simulink model "sampleModel2432_pp_1_1"  (R2018a)
settings: Solver=VariableStepAuto  StartTime=0.0  StopTime=10.0  RelTol=1e-3
undefined symbols (not defined in the file or in its folder): DiscIntNeverNeededParam, sigbuilder_block
libraries: simulink x293
(part 1 of 7)
settings Model: Creator=cyfuzz  LastModifiedBy=ishaf
settings CodeAppCC: StateflowObjectComments=on

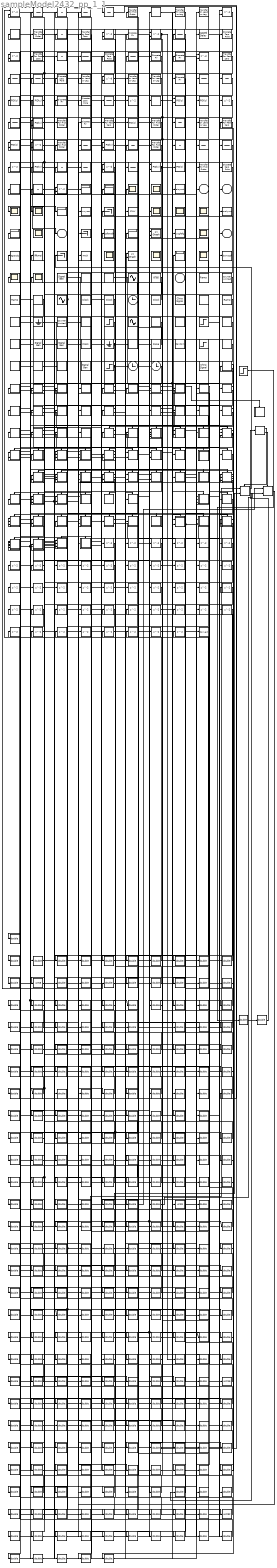
== system sampleModel2432_pp_1_1 ==
  cfblk128 : Inport
  cfblk{1,10,15,17,21,62,83} (7 alike) : Delay  ShowEnablePort=on  SampleTime=1
      settings: InputPortMap=u0,e6
  cfblk100 : ToWorkspace  VariableName=sxokymd  SaveFormat=Timeseries  SampleTime=-1
  cfblk{84..85,93,101,106,118} (6 alike) : Display
  cfblk{86..87,91..92,97..99,102,109,115,117,119,121..122} (14 alike) : Scope
      cfblk102 settings: Floating=on
      cfblk109 settings: Floating=on
      cfblk115 settings: Floating=on
      cfblk117 settings: Floating=on
      cfblk119 settings: Floating=on
      cfblk87 settings: Floating=on
      cfblk98 settings: Floating=on
      cfblk99 settings: Floating=on
  cfblk104 : Terminator
  cfblk105 : ToWorkspace  VariableName=zdioxsb  SaveFormat=Timeseries  SampleTime=-1
  cfblk107 : simulink/Sinks/XY Graph  xmin=-1  xmax=1  ymin=-1  ymax=1  st=-1
  cfblk108 : ToWorkspace  VariableName=yqgfefg  SaveFormat=Timeseries  SampleTime=-1
  cfblk11 : DiscreteStateSpace
  cfblk111 : ToWorkspace  VariableName=egcazdz  SaveFormat=Timeseries  SampleTime=-1
  cfblk112 : ToWorkspace  VariableName=iffcmsi  SaveFormat=Timeseries  SampleTime=-1
  cfblk113 : Terminator
  cfblk114 : ToFile  Filename=nxck  SaveFormat=Timeseries
  cfblk116 : simulink/Sinks/XY Graph  xmin=-1  xmax=1  ymin=-1  ymax=1  st=-1
  cfblk{6,12,53,57,63,67,79} (7 alike) : simulink/Discrete/Transfer Fcn First Order  PoleZ=0.95  ICPrevOutput=0.0  DoSatur=off
      settings: SourceProductName=Simulink
  cfblk120 : ToWorkspace  VariableName=bomsczf  SaveFormat=Timeseries  SampleTime=-1
  cfblk{123,152..153,164} (4 alike) : SignalGenerator  Units=rad/sec
  cfblk{124..125,132,139,147,163} (6 alike) : simulink/Sources/Repeating Sequence Interpolated  OutValues=[3 1 4 2 1].'  TimeValues=[0 0.1 0.5 0.6 1].'  LookUpMeth=Interpolation-Use End Values  tsamp=0.01  OutMin=[]  OutMax=[]  OutDataTypeStr=double  OutputDataTypeScalingMode=double  OutDataType=fixdt(0,8)  OutScaling=2^-10
  cfblk126 : Sin  SampleTime=0
  cfblk127 : Constant  Value=8785
  cfblk129 : simulink/Sources/Ramp  slope=1  start=0  InitialOutput=0
  cfblk{3,13,23,68,73,82} (6 alike) : UnitDelay
  cfblk130 : simulink/Sources/Counter Limited  uplimit=7  tsamp=-1
  cfblk131 : simulink/Sources/Ramp  slope=1  start=0  InitialOutput=0
  cfblk133 : Sin  SampleTime=0
  cfblk{134..135,137,154} (4 alike) : DigitalClock
  cfblk136 : Clock
  cfblk138 : simulink/Sources/Chirp Signal  f1=0.1  T=100  f2=1
  cfblk{14,22,30,55,60} (5 alike) : simulink/Discrete/Transfer Fcn Real Zero  ZeroZ=0.75  ICPrevInput=0.0  DoSatur=off
      settings: SourceProductName=Simulink  SourceProductBaseCode=SL
  cfblk140 : simulink/Sources/Ramp  slope=1  start=0  InitialOutput=0
  cfblk141 : Subsystem  Tag=STV Subsys  LoadFcn=sigbuilder_block('load');  StartFcn=sigbuilder_block('start');  StopFcn=sigbuilder_block('stop');  ClipboardFcn=sigbuilder_block('clipboard');  mask(Sigbuilder block){tuvar=[0:10]}
      mask help: Simulink:masks:SigbuilderBlock_MD
      mask init:
      | if ~strcmp(get_param(bdroot(gcbh),'SimulationStatus'),'stopped') tuvar = sigbuilder_block('maskInit'); end
      settings: CopyFcn=sigbuilder_block('copy');  DeleteFcn=sigbuilder_block('delete');  ModelCloseFcn=sigbuilder_block('modelClose');  PreSaveFcn=sigbuilder_block('preSave');  PauseFcn=sigbuilder_block('pause');  ContinueFcn=sigbuilder_block('continue');  NameChangeFcn=sigbuilder_block('namechange');  OpenFcn=sigbuilder_block('open',[437.6 199.2 550.4 400 ]);  CloseFcn=sigbuilder_block('close');
      mask Display: plot(0, 0, 100, 100,[2, 2, 32, 32, 2], [68, 8, 8, 68, 68],[32, 2], [38, 38], [32, 19, 2],[53, 60, 44], [32, 17, 17, 2],[16, 16, 31, 31]);txt = getActiveGroup(gcbh);text(2, 100, txt,'verticalAlignment', 'top');
  cfblk142 : Ground
  cfblk143 : simulink/Sources/Counter Limited  uplimit=7  tsamp=-1
  cfblk{144,150,160..161} (4 alike) : simulink/Sources/Repeating Sequence  rep_seq_t=[0 2]  rep_seq_y=[0 2]
  cfblk145 : Step  After=94  SampleTime=0
  cfblk146 : Sin  SampleTime=0
  cfblk148 : simulink/Sources/Repeating Sequence Stair  OutValues=[3 1 4 2 1].'  tsamp=-1  OutMin=[]  OutMax=[]  OutDataTypeStr=double  OutputDataTypeScalingMode=double  OutDataType=fixdt(0,8)  ConRadixGroup=Best Precision: Vector-wise  OutScaling=2^-12
  cfblk149 : Step  After=59  SampleTime=0
  cfblk151 : simulink/Sources/Band-Limited White Noise  Cov=[0.1]  Ts=0.1  seed=[23341]
  cfblk155 : Ground
  cfblk156 : Subsystem  Tag=STV Subsys  LoadFcn=sigbuilder_block('load');  StartFcn=sigbuilder_block('start');  StopFcn=sigbuilder_block('stop');  ClipboardFcn=sigbuilder_block('clipboard');  mask(Sigbuilder block){tuvar=[0:10]}
      mask help: Simulink:masks:SigbuilderBlock_MD
      mask init:
      | if ~strcmp(get_param(bdroot(gcbh),'SimulationStatus'),'stopped') tuvar = sigbuilder_block('maskInit'); end
      settings: CopyFcn=sigbuilder_block('copy');  DeleteFcn=sigbuilder_block('delete');  ModelCloseFcn=sigbuilder_block('modelClose');  PreSaveFcn=sigbuilder_block('preSave');  PauseFcn=sigbuilder_block('pause');  ContinueFcn=sigbuilder_block('continue');  NameChangeFcn=sigbuilder_block('namechange');  OpenFcn=sigbuilder_block('open',[437.6 199.2 550.4 400 ]);  CloseFcn=sigbuilder_block('close');
      mask Display: plot(0, 0, 100, 100,[2, 2, 32, 32, 2], [68, 8, 8, 68, 68],[32, 2], [38, 38], [32, 19, 2],[53, 60, 44], [32, 17, 17, 2],[16, 16, 31, 31]);txt = getActiveGroup(gcbh);text(2, 100, txt,'verticalAlignment', 'top');
  cfblk157 : DiscretePulseGenerator  PulseType=Time based  Period=10  PulseWidth=5
  cfblk158 : UniformRandomNumber  SampleTime=0.1
  cfblk159 : Step  After=53  SampleTime=0
  cfblk{16,27..28,38,43,54} (6 alike) : DiscreteFir  SampleTime=1
  cfblk162 : simulink/Sources/Counter Free-Running  NumBits=16  tsamp=-1
  cfblk165 : Step  After=66  SampleTime=0
  cfblk166 : Clock
  cfblk167 : Clock
  cfblk168 : Step  After=29  SampleTime=0
  cfblk169 : simulink/Sources/Chirp Signal  f1=0.1  T=100  f2=1
  cfblk{170..194} (25 alike) : If  SampleTime=1
  cfblk{2,18,51,64,70,74} (6 alike) : DiscreteTransferFcn  SampleTime=1
  cfblk19 : simulink/Discrete/Tapped Delay  vinit=0.0  samptime=-1  NumDelays=1  DelayOrder=Oldest  includeCurrent=off
  cfblk195 : Subsystem  TreatAsAtomicUnit=on
  cfblk196 : Subsystem  TreatAsAtomicUnit=on
  cfblk197 : Subsystem  TreatAsAtomicUnit=on
  cfblk198 : Subsystem  TreatAsAtomicUnit=on
  cfblk199 : Subsystem  TreatAsAtomicUnit=on
  cfblk{20,25,33,44,80} (5 alike) : DiscreteZeroPole  Poles=[0 0.5]  Gain=1
  cfblk200 : Subsystem  TreatAsAtomicUnit=on
  cfblk201 : Subsystem  TreatAsAtomicUnit=on
  cfblk202 : Subsystem  TreatAsAtomicUnit=on
  cfblk203 : Subsystem  TreatAsAtomicUnit=on
  cfblk204 : Subsystem  TreatAsAtomicUnit=on
  cfblk205 : Subsystem  TreatAsAtomicUnit=on
  cfblk206 : Subsystem  TreatAsAtomicUnit=on
  cfblk207 : Subsystem  TreatAsAtomicUnit=on
  cfblk208 : Subsystem  TreatAsAtomicUnit=on
  cfblk209 : Subsystem  TreatAsAtomicUnit=on
  cfblk210 : Subsystem  TreatAsAtomicUnit=on
  cfblk211 : Subsystem  TreatAsAtomicUnit=on
  cfblk212 : Subsystem  TreatAsAtomicUnit=on
  cfblk213 : Subsystem  TreatAsAtomicUnit=on
  cfblk214 : Subsystem  TreatAsAtomicUnit=on
  cfblk215 : Subsystem  TreatAsAtomicUnit=on
  cfblk216 : Subsystem  TreatAsAtomicUnit=on
  cfblk217 : Subsystem  TreatAsAtomicUnit=on
  cfblk218 : Subsystem  TreatAsAtomicUnit=on
  cfblk219 : Subsystem  TreatAsAtomicUnit=on
  cfblk220 : Subsystem  TreatAsAtomicUnit=on
  cfblk221 : Subsystem  TreatAsAtomicUnit=on
  cfblk222 : Subsystem  TreatAsAtomicUnit=on
  cfblk223 : Subsystem  TreatAsAtomicUnit=on
  cfblk224 : Subsystem  TreatAsAtomicUnit=on
  cfblk225 : Subsystem  TreatAsAtomicUnit=on
  cfblk226 : Subsystem  TreatAsAtomicUnit=on
  cfblk227 : Subsystem  TreatAsAtomicUnit=on
  cfblk228 : Subsystem  TreatAsAtomicUnit=on
  cfblk229 : Subsystem  TreatAsAtomicUnit=on
  cfblk230 : Subsystem  TreatAsAtomicUnit=on
  cfblk231 : Subsystem  TreatAsAtomicUnit=on
  cfblk232 : Subsystem  TreatAsAtomicUnit=on
  cfblk233 : Subsystem  TreatAsAtomicUnit=on
  cfblk234 : Subsystem  TreatAsAtomicUnit=on
  cfblk235 : Subsystem  TreatAsAtomicUnit=on
  cfblk236 : Subsystem  TreatAsAtomicUnit=on
  cfblk237 : Subsystem  TreatAsAtomicUnit=on
  cfblk238 : Subsystem  TreatAsAtomicUnit=on
  cfblk239 : Subsystem  TreatAsAtomicUnit=on
  cfblk{24,26,31..32,39,45,76} (7 alike) : DiscreteFilter  SampleTime=1
  cfblk240 : Subsystem  TreatAsAtomicUnit=on
  cfblk241 : Subsystem  TreatAsAtomicUnit=on
  cfblk242 : Subsystem  TreatAsAtomicUnit=on
  cfblk243 : Subsystem  TreatAsAtomicUnit=on
  cfblk244 : Subsystem  TreatAsAtomicUnit=on
  cfblk{46,50,71,245..288} (47 alike) : Delay  SampleTime=1
  cfblk289 : DataTypeConversion
  cfblk29 : Delay  DelayLengthSource=Input port  SampleTime=1
      settings: InputPortMap=u0,p1
  cfblk{8..9,34,36..37,59} (6 alike) : simulink/Discrete/Transfer Fcn Lead or Lag  PoleZ=0.95  ZeroZ=0.75  ICPrevOutput=0.0  ICPrevInput=0.0  DoSatur=off
      settings: SourceProductName=Simulink  SourceProductBaseCode=SL
  cfblk35 : Delay  DelayLengthSource=Input port  SampleTime=1
      settings: InputPortMap=u0,p1
  cfblk{4..5,40,58,66,69} (6 alike) : DiscreteIntegrator  ICPrevOutput=DiscIntNeverNeededParam  ICPrevScaledInput=DiscIntNeverNeededParam
  cfblk{41..42,49,56,72,78} (6 alike) : simulink/Continuous/PID Controller  Controller=PID  TimeDomain=Discrete-time  SampleTime=1  IntegratorMethod=Forward Euler  FilterMethod=Forward Euler  Form=Parallel  UseFilter=on  ControllerParametersSource=internal  P=1  I=1  D=0  N=100  InitialConditionSource=internal  InitialConditionForIntegrator=0  InitialConditionForFilter=0  ExternalReset=none  LimitOutput=off  UpperSaturationLimit=inf  LowerSaturationLimit=-inf  LinearizeAsGain=off  AntiWindupMode=none  Kb=1  TrackingMode=off  Kt=1  PParamMin=[]  PParamMax=[]  IParamMin=[]  IParamMax=[]  DParamMin=[]  DParamMax=[]  NParamMin=[]  NParamMax=[]  KbParamMin=[]  KbParamMax=[]  KtParamMin=[]  KtParamMax=[]  POutMin=[]  POutMax=[]  IOutMin=[]  IOutMax=[]  DOutMin=[]  DOutMax=[]  NOutMin=[]  NOutMax=[]  KbOutMin=[]  KbOutMax=[]  KtOutMin=[]  KtOutMax=[]  IntegratorOutMin=[]  IntegratorOutMax=[]  FilterOutMin=[]  FilterOutMax=[]  SumOutMin=[]  SumOutMax=[]  SumI1OutMin=[]  SumI1OutMax=[]  SumI2OutMin=[]  SumI2OutMax=[]  SumI3OutMin=[]  SumI3OutMax=[]  SumDOutMin=[]  SumDOutMax=[]  SaturationOutMin=[]  SaturationOutMax=[]  IntegratorContinuousStateAttributes=''  IntegratorStateMustResolveToSignalObject=off  IntegratorRTWStateStorageClass=Auto  FilterContinuousStateAttributes=''  FilterStateMustResolveToSignalObject=off  FilterRTWStateStorageClass=Auto  DifferentiatorICPrevScaledInput=0  DifferentiatorOutMin=[]  DifferentiatorOutMax=[]  FilterDiffOutCoefMin=[]  FilterDiffOutCoefMax=[]  SumDenOutMin=[]  SumDenOutMax=[]  SumNumOutMin=[]  SumNumOutMax=[]  ReciprocalOutMin=[]  ReciprocalOutMax=[]  DivideOutMin=[]  DivideOutMax=[]  TunerSelectOption=Transfer Function Based (PID Tuner App)
  cfblk47 : DiscreteStateSpace
  cfblk{48,52,61,65,77} (5 alike) : simulink/Continuous/PID Controller (2DOF)  Controller=PID  TimeDomain=Discrete-time  SampleTime=1  IntegratorMethod=Forward Euler  FilterMethod=Forward Euler  Form=Parallel  UseFilter=on  ControllerParametersSource=internal  P=1  I=1  D=0  N=100  b=1  c=1  InitialConditionSource=internal  InitialConditionForIntegrator=0  InitialConditionForFilter=0  ExternalReset=none  LimitOutput=off  UpperSaturationLimit=inf  LowerSaturationLimit=-inf  LinearizeAsGain=off  AntiWindupMode=none  Kb=1  TrackingMode=off  Kt=1  PParamMin=[]  PParamMax=[]  IParamMin=[]  IParamMax=[]  DParamMin=[]  DParamMax=[]  NParamMin=[]  NParamMax=[]  bParamMin=[]  bParamMax=[]  cParamMin=[]  cParamMax=[]  KbParamMin=[]  KbParamMax=[]  KtParamMin=[]  KtParamMax=[]  POutMin=[]  POutMax=[]  IOutMin=[]  IOutMax=[]  DOutMin=[]  DOutMax=[]  NOutMin=[]  NOutMax=[]  bOutMin=[]  bOutMax=[]  cOutMin=[]  cOutMax=[]  KbOutMin=[]  KbOutMax=[]  KtOutMin=[]  KtOutMax=[]  IntegratorOutMin=[]  IntegratorOutMax=[]  FilterOutMin=[]  FilterOutMax=[]  SumOutMin=[]  SumOutMax=[]  Sum1OutMin=[]  Sum1OutMax=[]  Sum2OutMin=[]  Sum2OutMax=[]  Sum3OutMin=[]  Sum3OutMax=[]  SumI1OutMin=[]  SumI1OutMax=[]  SumI2OutMin=[]  SumI2OutMax=[]  SumI3OutMin=[]  SumI3OutMax=[]  SumDOutMin=[]  SumDOutMax=[]  SaturationOutMin=[]  SaturationOutMax=[]  IntegratorContinuousStateAttributes=''  IntegratorStateMustResolveToSignalObject=off  IntegratorRTWStateStorageClass=Auto  FilterContinuousStateAttributes=''  FilterStateMustResolveToSignalObject=off  FilterRTWStateStorageClass=Auto  DifferentiatorICPrevScaledInput=0  DifferentiatorOutMin=[]  DifferentiatorOutMax=[]  FilterDiffOutCoefMin=[]  FilterDiffOutCoefMax=[]  SumDenOutMin=[]  SumDenOutMax=[]  SumNumOutMin=[]  SumNumOutMax=[]  ReciprocalOutMin=[]  ReciprocalOutMax=[]  DivideOutMin=[]  DivideOutMax=[]  TunerSelectOption=Transfer Function Based (PID Tuner App)
  cfblk7 : simulink/Discrete/Difference  ICPrevInput=0.0  OutMin=[]  OutMax=[]  OutDataTypeStr=Inherit: Inherit via back propagation  OutDataType=fixdt(1, 16)  OutScaling=2^-10  DoSatur=off
  cfblk75 : Delay  DelayLengthSource=Input port  SampleTime=1
      settings: InputPortMap=u0,p1
  cfblk81 : simulink/Discrete/Difference  ICPrevInput=0.0  OutMin=[]  OutMax=[]  OutDataTypeStr=Inherit: Inherit via back propagation  OutDataType=fixdt(1, 16)  OutScaling=2^-10  DoSatur=off
  cfblk88 : ToWorkspace  VariableName=eizyzmt  SaveFormat=Timeseries  SampleTime=-1
  cfblk94 : ToWorkspace  VariableName=uvxysss  SaveFormat=Timeseries  SampleTime=-1
  cfblk95 : Terminator
  cfblk96 : ToFile  Filename=clwv  SaveFormat=Timeseries
  cyemi_{0..11,13..47,55,89..92,142..143,194,205..209,216..217,227,290..292,305..307,334,339..340,377..378,386,393,395..397,432..433,438..439,446..448,453..454,462..463,474..475,487..488,495,588..590,620..623,634,643..645,650..651,658,695..697,738,755..756,792..793,800..801,813..814,847..849,875..876,883,898..899,925,935,949..950,1002..1003,1017..1018,1084..1086,1092..1096,1105,1175..1177,1255,1296..1343,1345..1403,1405..1419} (272 alike) : DataTypeConversion  OutDataTypeStr=double
  cyemi_12 : DataTypeConversion  OutDataTypeStr=uint8
  cyemi_1344 : DataTypeConversion  OutDataTypeStr=uint16
  cyemi_1404 : DataTypeConversion  OutDataTypeStr=uint32
  cyemi_799 : DataTypeConversion  OutDataTypeStr=uint8
  cfblk89 : Outport
  cfblk90 : Outport  Port=2
  cfblk103 : Outport  Port=3
  cfblk110 : Outport  Port=4
  wires:
  cfblk69/1 -> cyemi_1315/1, cyemi_1326/1
  cfblk137/1 -> cfblk116/1
  cfblk136/1 -> cfblk121/1, cyemi_474/1
  cfblk16/1 -> cyemi_216/1, cyemi_800/1
  cfblk165/1 -> cyemi_207/1, cyemi_1363/1, cyemi_755/1
  cfblk41/1 -> cfblk93/1
  cfblk199/1(cfblk2) -> cfblk85/1
  cfblk58/1 -> cfblk107/1, cyemi_756/1
  cfblk149/1 -> cfblk90/1
  cfblk227/1(cfblk2) -> cfblk113/1
  cfblk71/1 -> cfblk103/1
  cfblk73/1 -> cfblk104/1
  cfblk34/1 -> cyemi_623/1, cyemi_1366/1
  cfblk129/1 -> cfblk107/2
  cfblk208/1(cfblk2) -> cfblk118/1
  cfblk133/1 -> cyemi_92/1, cyemi_738/1
  cfblk48/1 -> cyemi_305/1, cyemi_1365/1
  cfblk223/1(cfblk2) -> cfblk110/1
  cfblk29/1 -> cyemi_1385/1, cyemi_1396/1
  cfblk77/1 -> cyemi_1307/1, cyemi_1397/1, cyemi_1354/1
  cfblk9/1 -> cfblk92/1
  cfblk213/2(cfblk9) -> cyemi_217/1, cyemi_697/1
  cfblk204/1(cfblk2) -> cfblk101/1
  cfblk202/2(cfblk9) -> cfblk122/1
  cfblk157/1 -> cfblk106/1
  cfblk57/1 -> cfblk116/2
  cfblk17/1 -> cfblk91/1, cyemi_1332/1
  cfblk241/2(cfblk12) -> cfblk84/1, cyemi_1341/1
  cfblk205/3(cfblk8) -> cfblk89/1
  cfblk44/1 -> cyemi_11/1, cyemi_793/1
  cfblk155/1 -> cyemi_801/1, cyemi_1415/1
  cfblk200/2(cfblk10) -> cyemi_1306/1, cyemi_1384/1
  cfblk226/1(cfblk2) -> cfblk97/1
  cfblk238/4(cfblk15) -> cyemi_695/1, cyemi_925/1
  cfblk231/2(cfblk13) -> cyemi_26/1, cyemi_1340/1
  cfblk222/2(cfblk8) -> cfblk86/1, cyemi_848/1
  cfblk220/3(cfblk13) -> cfblk95/1
  cfblk170/1 -> cfblk195/Action
  cfblk170/2 -> cfblk196/Action
  cfblk171/1 -> cfblk197/Action
  cfblk171/2 -> cfblk198/Action
  cfblk172/1 -> cfblk199/Action
  cfblk172/2 -> cfblk200/Action
  cfblk173/1 -> cfblk201/Action
  cfblk173/2 -> cfblk202/Action
  cfblk174/1 -> cfblk203/Action
  cfblk174/2 -> cfblk204/Action
  cfblk175/1 -> cfblk205/Action
  cfblk175/2 -> cfblk206/Action
  cfblk176/1 -> cfblk207/Action
  cfblk176/2 -> cfblk208/Action
  cfblk177/1 -> cfblk209/Action
  cfblk177/2 -> cfblk210/Action
  cfblk178/1 -> cfblk211/Action
  cfblk178/2 -> cfblk212/Action
  cfblk179/1 -> cfblk213/Action
  cfblk179/2 -> cfblk214/Action
  cfblk180/1 -> cfblk215/Action
  cfblk180/2 -> cfblk216/Action
  cfblk181/1 -> cfblk217/Action
  cfblk181/2 -> cfblk218/Action
  cfblk182/1 -> cfblk219/Action
  cfblk182/2 -> cfblk220/Action
  cfblk183/1 -> cfblk221/Action
  cfblk183/2 -> cfblk222/Action
  cfblk184/1 -> cfblk223/Action
  cfblk184/2 -> cfblk224/Action
  cfblk185/1 -> cfblk225/Action
  cfblk185/2 -> cfblk226/Action
  cfblk186/1 -> cfblk227/Action
  cfblk186/2 -> cfblk228/Action
  cfblk187/1 -> cfblk229/Action
  cfblk187/2 -> cfblk230/Action
  cfblk188/1 -> cfblk231/Action
  cfblk188/2 -> cfblk232/Action
  cfblk189/1 -> cfblk233/Action
  cfblk189/2 -> cfblk234/Action
  cfblk190/1 -> cfblk235/Action
  cfblk190/2 -> cfblk236/Action
  cfblk191/1 -> cfblk237/Action
  cfblk191/2 -> cfblk238/Action
  cfblk192/1 -> cfblk239/Action
  cfblk192/2 -> cfblk240/Action
  cfblk193/1 -> cfblk241/Action
  cfblk193/2 -> cfblk242/Action
  cfblk194/1 -> cfblk243/Action
  cfblk194/2 -> cfblk244/Action
  cyemi_0/1 -> cfblk1/1
  cfblk158/1 -> cyemi_0/1
  cyemi_1/1 -> cfblk1/2
  cfblk232/1(cfblk2) -> cyemi_1/1
  cyemi_2/1 -> cfblk10/1
  cfblk231/1(cfblk2) -> cyemi_2/1
  cyemi_3/1 -> cfblk10/2
  cfblk196/1(cfblk2) -> cyemi_3/1
  cyemi_4/1 -> cfblk100/1
  cfblk68/1 -> cyemi_4/1
  cyemi_5/1 -> cfblk105/1
  cfblk205/2(cfblk7) -> cyemi_5/1
  cyemi_6/1 -> cfblk108/1
  cfblk139/1 -> cyemi_6/1
  cyemi_7/1 -> cfblk11/1
  cfblk52/1 -> cyemi_7/1
  cyemi_8/1 -> cfblk111/1
  cfblk15/1 -> cyemi_8/1
  cyemi_9/1 -> cfblk112/1
  cfblk204/2(cfblk11) -> cyemi_9/1
  cyemi_10/1 -> cfblk114/1
  cfblk229/1(cfblk2) -> cyemi_10/1
  cyemi_11/1 -> cfblk12/1
  cyemi_12/1 -> cfblk120/1
  cfblk130/1 -> cyemi_12/1
  cyemi_13/1 -> cfblk13/1
  cfblk151/1 -> cyemi_13/1
  cyemi_14/1 -> cfblk14/1
  cfblk223/2(cfblk9) -> cyemi_14/1
  cyemi_15/1 -> cfblk15/1
  cfblk4/1 -> cyemi_15/1
  cyemi_16/1 -> cfblk15/2
  cfblk27/1 -> cyemi_16/1
  cyemi_17/1 -> cfblk16/1
  cfblk64/1 -> cyemi_17/1
  cyemi_18/1 -> cfblk17/1
  cfblk39/1 -> cyemi_18/1
  cyemi_19/1 -> cfblk17/2
  cfblk82/1 -> cyemi_19/1
  cyemi_20/1 -> cfblk170/1
  cfblk166/1 -> cyemi_20/1
  cyemi_21/1 -> cfblk171/1
  cfblk145/1 -> cyemi_21/1
  cyemi_22/1 -> cfblk172/1
  cfblk269/1 -> cyemi_22/1
  cyemi_23/1 -> cfblk173/1
  cfblk263/1 -> cyemi_23/1
  cyemi_24/1 -> cfblk174/1
  cfblk279/1 -> cyemi_24/1
  cyemi_25/1 -> cfblk175/1
  cfblk150/1 -> cyemi_25/1
  cyemi_26/1 -> cfblk176/1
  cyemi_27/1 -> cfblk177/1
  cfblk249/1 -> cyemi_27/1
  cyemi_28/1 -> cfblk178/1
  cfblk216/2(cfblk14) -> cyemi_28/1
  cyemi_29/1 -> cfblk179/1
  cfblk288/1 -> cyemi_29/1
  cyemi_30/1 -> cfblk18/1
  cfblk66/1 -> cyemi_30/1
  cyemi_31/1 -> cfblk180/1
  cfblk132/1 -> cyemi_31/1
  cyemi_32/1 -> cfblk181/1
  cfblk202/1(cfblk2) -> cyemi_32/1
  cyemi_33/1 -> cfblk182/1
  cfblk243/1(cfblk2) -> cyemi_33/1
  cyemi_34/1 -> cfblk183/1
  cfblk261/1 -> cyemi_34/1
  cyemi_35/1 -> cfblk184/1
  cfblk220/2(cfblk12) -> cyemi_35/1
  cyemi_36/1 -> cfblk185/1
  cfblk215/2(cfblk11) -> cyemi_36/1
  cyemi_37/1 -> cfblk186/1
  cyemi_38/1 -> cfblk187/1
  cfblk154/1 -> cyemi_38/1
  cyemi_39/1 -> cfblk188/1
  cfblk153/1 -> cyemi_39/1
  cyemi_40/1 -> cfblk189/1
  cfblk55/1 -> cyemi_40/1
  cyemi_41/1 -> cfblk19/1
  cfblk146/1 -> cyemi_41/1
  cyemi_42/1 -> cfblk190/1
  cfblk37/1 -> cyemi_42/1
  cyemi_43/1 -> cfblk191/1
  cfblk256/1 -> cyemi_43/1
  cyemi_44/1 -> cfblk192/1
  cfblk275/1 -> cyemi_44/1
  cyemi_45/1 -> cfblk193/1
  cfblk33/1 -> cyemi_45/1
  cyemi_46/1 -> cfblk194/1
  cfblk274/1 -> cyemi_46/1
  cyemi_47/1 -> cfblk195/1(cfblk1)
  cfblk242/2(cfblk14) -> cyemi_47/1
  cyemi_55/1 -> cfblk196/1(cfblk1)
  cfblk24/1 -> cyemi_55/1
  cyemi_89/1 -> cfblk197/1(cfblk1)
  cfblk233/1(cfblk2) -> cyemi_89/1
  cyemi_90/1 -> cfblk197/2(cfblk14)
  cfblk47/1 -> cyemi_90/1
  cyemi_91/1 -> cfblk197/3(cfblk15)
  cfblk163/1 -> cyemi_91/1
  cyemi_92/1 -> cfblk197/4(cfblk16)
  cyemi_142/1 -> cfblk198/1(cfblk1)
  cfblk148/1 -> cyemi_142/1
  cyemi_143/1 -> cfblk198/2(cfblk11)
  cfblk267/1 -> cyemi_143/1
  cyemi_194/1 -> cfblk199/1(cfblk1)
  cfblk210/1(cfblk2) -> cyemi_194/1
  cyemi_205/1 -> cfblk2/1
  cfblk78/1 -> cyemi_205/1
  cyemi_206/1 -> cfblk20/1
  cfblk38/1 -> cyemi_206/1
  cyemi_207/1 -> cfblk200/1(cfblk1)
  cyemi_208/1 -> cfblk200/2(cfblk8)
  cfblk251/1 -> cyemi_208/1
  cyemi_209/1 -> cfblk200/3(cfblk9)
  cfblk271/1 -> cyemi_209/1
  cyemi_216/1 -> cfblk201/1(cfblk1)
  cyemi_217/1 -> cfblk201/2(cfblk11)
  cyemi_227/1 -> cfblk202/1(cfblk1)
  cfblk282/1 -> cyemi_227/1
  cyemi_290/1 -> cfblk203/1(cfblk1)
  cfblk43/1 -> cyemi_290/1
  cyemi_291/1 -> cfblk203/2(cfblk13)
  cfblk273/1 -> cyemi_291/1
  cyemi_292/1 -> cfblk203/3(cfblk14)
  cfblk18/1 -> cyemi_292/1
  cyemi_305/1 -> cfblk204/1(cfblk1)
  cyemi_306/1 -> cfblk204/2(cfblk9)
  cfblk287/1 -> cyemi_306/1
  cyemi_307/1 -> cfblk204/3(cfblk10)
  cfblk28/1 -> cyemi_307/1
  cyemi_334/1 -> cfblk205/1(cfblk1)
  cfblk5/1 -> cyemi_334/1
  cyemi_339/1 -> cfblk206/1(cfblk1)
  cfblk63/1 -> cyemi_339/1
  cyemi_340/1 -> cfblk206/2(cfblk10)
  cfblk245/1 -> cyemi_340/1
  cyemi_377/1 -> cfblk207/1(cfblk1)
  cfblk124/1 -> cyemi_377/1
  cyemi_378/1 -> cfblk207/2(cfblk8)
  cfblk203/3(cfblk16) -> cyemi_378/1
  cyemi_386/1 -> cfblk208/1(cfblk1)
  cfblk161/1 -> cyemi_386/1
  cfblk214/1(cfblk2) -> cyemi_393/1
  cyemi_395/1 -> cfblk21/1
  cfblk11/1 -> cyemi_395/1
  cyemi_396/1 -> cfblk21/2
  cfblk70/1 -> cyemi_396/1
  cyemi_397/1 -> cfblk210/1(cfblk1)
  cfblk250/1 -> cyemi_397/1
  cfblk168/1 -> cyemi_432/1
  cfblk226/2(cfblk14) -> cyemi_433/1
  cyemi_438/1 -> cfblk212/1(cfblk1)
  cfblk208/3(cfblk8) -> cyemi_438/1
  cyemi_439/1 -> cfblk212/2(cfblk9)
  cfblk147/1 -> cyemi_439/1
  cyemi_446/1 -> cfblk213/1(cfblk1)
  cfblk283/1 -> cyemi_446/1
  cyemi_447/1 -> cfblk213/2(cfblk7)
  cfblk270/1 -> cyemi_447/1
  cyemi_448/1 -> cfblk213/3(cfblk8)
  cfblk254/1 -> cyemi_448/1
  cyemi_453/1 -> cfblk214/1(cfblk1)
  cfblk206/1(cfblk2) -> cyemi_453/1
  cyemi_454/1 -> cfblk214/2(cfblk9)
  cfblk169/1 -> cyemi_454/1
  cyemi_462/1 -> cfblk215/1(cfblk1)
  cfblk264/1 -> cyemi_462/1
  cyemi_463/1 -> cfblk215/2(cfblk10)
  cfblk201/1(cfblk2) -> cyemi_463/1
  cyemi_474/1 -> cfblk216/1(cfblk1)
  cyemi_475/1 -> cfblk216/2(cfblk13)
  cfblk255/1 -> cyemi_475/1
  cyemi_487/1 -> cfblk217/1(cfblk1)
  cfblk266/1 -> cyemi_487/1
  cyemi_488/1 -> cfblk217/2(cfblk7)
  cfblk268/1 -> cyemi_488/1
  cyemi_495/1 -> cfblk218/1(cfblk1)
  cfblk54/1 -> cyemi_495/1
  cfblk127/1 -> cyemi_588/1
  cfblk286/1 -> cyemi_589/1
  cfblk285/1 -> cyemi_590/1
  cyemi_620/1 -> cfblk22/1
  cfblk198/1(cfblk2) -> cyemi_620/1
  cyemi_621/1 -> cfblk220/1(cfblk1)
  cfblk277/1 -> cyemi_621/1
  cyemi_622/1 -> cfblk220/2(cfblk10)
  cfblk281/1 -> cyemi_622/1
  cyemi_623/1 -> cfblk220/3(cfblk11)
  cyemi_634/1 -> cfblk221/1(cfblk1)
  cyemi_643/1 -> cfblk222/1(cfblk1)
  cfblk128/1 -> cyemi_643/1
  cyemi_644/1 -> cfblk222/2(cfblk6)
  cfblk260/1 -> cyemi_644/1
  cyemi_645/1 -> cfblk222/3(cfblk7)
  cfblk247/1 -> cyemi_645/1
  cyemi_650/1 -> cfblk223/1(cfblk1)
  cfblk134/1 -> cyemi_650/1
  cyemi_651/1 -> cfblk223/2(cfblk8)
  cfblk212/3(cfblk11) -> cyemi_651/1
  cfblk207/1(cfblk2) -> cyemi_658/1
  cfblk272/1 -> cyemi_696/1
  cyemi_738/1 -> cfblk226/1(cfblk1)
  cyemi_755/1 -> cfblk227/1(cfblk1)
  cyemi_756/1 -> cfblk227/2(cfblk11)
  cyemi_792/1 -> cfblk228/1(cfblk1)
  cfblk159/1 -> cyemi_792/1
  cyemi_793/1 -> cfblk228/2(cfblk8)
  cyemi_799/1 -> cfblk229/1(cfblk1)
  cfblk143/1 -> cyemi_799/1
  cyemi_800/1 -> cfblk229/2(cfblk12)
  cyemi_801/1 -> cfblk229/3(cfblk13)
  cyemi_813/1 -> cfblk23/1
  cfblk197/1(cfblk2) -> cyemi_813/1
  cyemi_814/1 -> cfblk230/1(cfblk1)
  cfblk215/3(cfblk12) -> cyemi_814/1
  cyemi_847/1 -> cfblk231/1(cfblk1)
  cfblk6/1 -> cyemi_847/1
  cyemi_848/1 -> cfblk231/2(cfblk11)
  cyemi_849/1 -> cfblk231/3(cfblk12)
  cfblk278/1 -> cyemi_849/1
  cyemi_875/1 -> cfblk232/1(cfblk1)
  cfblk280/1 -> cyemi_875/1
  cyemi_876/1 -> cfblk232/2(cfblk7)
  cfblk222/1(cfblk2) -> cyemi_876/1
  cyemi_883/1 -> cfblk233/1(cfblk1)
  cfblk262/1 -> cyemi_883/1
  cyemi_898/1 -> cfblk234/1(cfblk1)
  cfblk257/1 -> cyemi_898/1
  cyemi_899/1 -> cfblk234/2(cfblk7)
  cyemi_925/1 -> cfblk235/1(cfblk1)
  cyemi_935/1 -> cfblk236/1(cfblk1)
  cfblk81/1 -> cyemi_935/1
  cfblk25/1 -> cyemi_949/1
  cfblk259/1 -> cyemi_950/1
  cyemi_1002/1 -> cfblk238/1(cfblk1)
  cfblk123/1 -> cyemi_1002/1
  cyemi_1003/1 -> cfblk238/2(cfblk12)
  cfblk152/1 -> cyemi_1003/1
  cyemi_1017/1 -> cfblk239/1(cfblk1)
  cfblk138/1 -> cyemi_1017/1
  cyemi_1018/1 -> cfblk239/2(cfblk10)
  cfblk265/1 -> cyemi_1018/1
  cyemi_1084/1 -> cfblk24/1
  cfblk45/1 -> cyemi_1084/1
  cyemi_1085/1 -> cfblk240/1(cfblk1)
  cyemi_1086/1 -> cfblk240/2(cfblk7)
  cfblk205/1(cfblk2) -> cyemi_1086/1
  cyemi_1092/1 -> cfblk241/1(cfblk1)
  cfblk252/1 -> cyemi_1092/1
  cyemi_1093/1 -> cfblk241/2(cfblk8)
  cfblk276/1 -> cyemi_1093/1
  cyemi_1094/1 -> cfblk241/3(cfblk9)
  cfblk215/1(cfblk2) -> cyemi_1094/1
  cyemi_1095/1 -> cfblk241/4(cfblk10)
  cfblk258/1 -> cyemi_1095/1
  cyemi_1096/1 -> cfblk241/5(cfblk11)
  cfblk284/1 -> cyemi_1096/1
  cyemi_1105/1 -> cfblk242/1(cfblk1)
  cfblk248/1 -> cyemi_1105/1
  cyemi_1175/1 -> cfblk243/1(cfblk1)
  cfblk246/1 -> cyemi_1175/1
  cyemi_1176/1 -> cfblk243/2(cfblk11)
  cfblk234/1(cfblk2) -> cyemi_1176/1
  cyemi_1177/1 -> cfblk243/3(cfblk12)
  cfblk253/1 -> cyemi_1177/1
  cyemi_1255/1 -> cfblk244/1(cfblk1)
  cfblk144/1 -> cyemi_1255/1
  cyemi_1296/1 -> cfblk245/1
  cyemi_1297/1 -> cfblk246/1
  cfblk213/1(cfblk2) -> cyemi_1297/1
  cyemi_1298/1 -> cfblk247/1
  cfblk241/1(cfblk2) -> cyemi_1298/1
  cyemi_1299/1 -> cfblk248/1
  cfblk10/1 -> cyemi_1299/1
  cyemi_1300/1 -> cfblk249/1
  cfblk20/1 -> cyemi_1300/1
  cyemi_1301/1 -> cfblk25/1
  cfblk221/1(cfblk2) -> cyemi_1301/1
  cyemi_1302/1 -> cfblk250/1
  cfblk7/1 -> cyemi_1302/1
  cyemi_1303/1 -> cfblk251/1
  cfblk65/1 -> cyemi_1303/1
  cyemi_1304/1 -> cfblk252/1
  cfblk200/1(cfblk2) -> cyemi_1304/1
  cyemi_1305/1 -> cfblk253/1
  cfblk60/1 -> cyemi_1305/1
  cyemi_1306/1 -> cfblk254/1
  cyemi_1307/1 -> cfblk255/1
  cyemi_1308/1 -> cfblk256/1
  cfblk51/1 -> cyemi_1308/1
  cyemi_1309/1 -> cfblk257/1
  cfblk238/2(cfblk13) -> cyemi_1309/1
  cyemi_1310/1 -> cfblk258/1
  cfblk238/3(cfblk14) -> cyemi_1310/1
  cyemi_1311/1 -> cfblk259/1
  cfblk235/1(cfblk2) -> cyemi_1311/1
  cyemi_1312/1 -> cfblk26/1
  cfblk35/1 -> cyemi_1312/1
  cyemi_1313/1 -> cfblk260/1
  cfblk235/2(cfblk8) -> cyemi_1313/1
  cyemi_1314/1 -> cfblk261/1
  cfblk61/1 -> cyemi_1314/1
  cyemi_1315/1 -> cfblk262/1
  cyemi_1316/1 -> cfblk263/1
  cfblk8/1 -> cyemi_1316/1
  cyemi_1317/1 -> cfblk264/1
  cfblk30/1 -> cyemi_1317/1
  cyemi_1318/1 -> cfblk265/1
  cfblk76/1 -> cyemi_1318/1
  cyemi_1319/1 -> cfblk266/1
  cfblk239/1(cfblk2) -> cyemi_1319/1
  cyemi_1320/1 -> cfblk267/1
  cfblk239/2(cfblk11) -> cyemi_1320/1
  cyemi_1321/1 -> cfblk268/1
  cfblk22/1 -> cyemi_1321/1
  cyemi_1322/1 -> cfblk269/1
  cfblk198/2(cfblk12) -> cyemi_1322/1
  cyemi_1323/1 -> cfblk27/1
  cyemi_1324/1 -> cfblk270/1
  cfblk218/2(cfblk16) -> cyemi_1324/1
  cyemi_1325/1 -> cfblk271/1
  cfblk236/1(cfblk2) -> cyemi_1325/1
  cyemi_1326/1 -> cfblk272/1
  cyemi_1327/1 -> cfblk273/1
  cfblk49/1 -> cyemi_1327/1
  cyemi_1328/1 -> cfblk274/1
  cfblk203/1(cfblk2) -> cyemi_1328/1
  cyemi_1329/1 -> cfblk275/1
  cfblk244/2(cfblk7) -> cyemi_1329/1
  cyemi_1330/1 -> cfblk276/1
  cfblk67/1 -> cyemi_1330/1
  cyemi_1331/1 -> cfblk277/1
  cfblk207/2(cfblk9) -> cyemi_1331/1
  cyemi_1332/1 -> cfblk278/1
  cyemi_1333/1 -> cfblk279/1
  cfblk220/4(cfblk14) -> cyemi_1333/1
  cyemi_1334/1 -> cfblk28/1
  cyemi_1335/1 -> cfblk280/1
  cfblk40/1 -> cyemi_1335/1
  cyemi_1336/1 -> cfblk281/1
  cfblk212/4(cfblk12) -> cyemi_1336/1
  cyemi_1337/1 -> cfblk282/1
  cfblk195/1(cfblk2) -> cyemi_1337/1
  cyemi_1338/1 -> cfblk283/1
  cfblk74/1 -> cyemi_1338/1
  cyemi_1339/1 -> cfblk284/1
  cfblk242/5(cfblk17) -> cyemi_1339/1
  cyemi_1340/1 -> cfblk285/1
  cyemi_1341/1 -> cfblk286/1
  cyemi_1342/1 -> cfblk287/1
  cfblk56/1 -> cyemi_1342/1
  cyemi_1343/1 -> cfblk288/1
  cfblk204/3(cfblk12) -> cyemi_1343/1
  cyemi_1344/1 -> cfblk289/1
  cfblk162/1 -> cyemi_1344/1
  cyemi_1345/1 -> cfblk29/1
  cfblk240/1(cfblk2) -> cyemi_1345/1
  cyemi_1346/1 -> cfblk29/2
  cfblk126/1 -> cyemi_1346/1
  cyemi_1347/1 -> cfblk3/1
  cfblk226/3(cfblk15) -> cyemi_1347/1
  cyemi_1348/1 -> cfblk30/1
  cfblk31/1 -> cyemi_1348/1
  cyemi_1349/1 -> cfblk31/1
  cfblk62/1 -> cyemi_1349/1
  cyemi_1350/1 -> cfblk32/1
  cfblk212/2(cfblk10) -> cyemi_1350/1
  cyemi_1351/1 -> cfblk33/1
  cfblk289/1 -> cyemi_1351/1
  cyemi_1352/1 -> cfblk34/1
  cfblk125/1 -> cyemi_1352/1
  cyemi_1353/1 -> cfblk35/1
  cyemi_1354/1 -> cfblk35/2
  cyemi_1355/1 -> cfblk36/1
  cfblk53/1 -> cyemi_1355/1
  cyemi_1356/1 -> cfblk37/1
  cfblk42/1 -> cyemi_1356/1
  cyemi_1357/1 -> cfblk38/1
  cfblk242/1(cfblk2) -> cyemi_1357/1
  cyemi_1358/1 -> cfblk39/1
  cfblk14/1 -> cyemi_1358/1
  cyemi_1359/1 -> cfblk4/1
  cfblk238/1(cfblk2) -> cyemi_1359/1
  cyemi_1360/1 -> cfblk40/1
  cfblk212/1(cfblk2) -> cyemi_1360/1
  cyemi_1361/1 -> cfblk41/1
  cfblk242/4(cfblk16) -> cyemi_1361/1
  cyemi_1362/1 -> cfblk42/1
  cfblk244/1(cfblk2) -> cyemi_1362/1
  cyemi_1363/1 -> cfblk43/1
  cyemi_1364/1 -> cfblk44/1
  cfblk195/2(cfblk7) -> cyemi_1364/1
  cyemi_1365/1 -> cfblk45/1
  cyemi_1366/1 -> cfblk46/1
  cyemi_1367/1 -> cfblk47/1
  cfblk167/1 -> cyemi_1367/1
  cyemi_1368/1 -> cfblk48/1
  cfblk75/1 -> cyemi_1368/1
  cyemi_1369/1 -> cfblk48/2
  cyemi_1370/1 -> cfblk49/1
  cfblk240/2(cfblk8) -> cyemi_1370/1
  cyemi_1371/1 -> cfblk5/1
  cfblk160/1 -> cyemi_1371/1
  cyemi_1372/1 -> cfblk50/1
  cfblk230/1(cfblk2) -> cyemi_1372/1
  cyemi_1373/1 -> cfblk51/1
  cfblk216/1(cfblk2) -> cyemi_1373/1
  cyemi_1374/1 -> cfblk52/1
  cfblk218/1(cfblk2) -> cyemi_1374/1
  cyemi_1375/1 -> cfblk52/2
  cyemi_1376/1 -> cfblk53/1
  cfblk46/1 -> cyemi_1376/1
  cyemi_1377/1 -> cfblk54/1
  cfblk36/1 -> cyemi_1377/1
  cyemi_1378/1 -> cfblk55/1
  cfblk164/1 -> cyemi_1378/1
  cyemi_1379/1 -> cfblk56/1
  cfblk50/1 -> cyemi_1379/1
  cyemi_1380/1 -> cfblk57/1
  cfblk3/1 -> cyemi_1380/1
  cyemi_1381/1 -> cfblk58/1
  cfblk26/1 -> cyemi_1381/1
  cyemi_1382/1 -> cfblk59/1
  cfblk199/2(cfblk11) -> cyemi_1382/1
  cyemi_1383/1 -> cfblk6/1
  cfblk229/2(cfblk14) -> cyemi_1383/1
  cyemi_1384/1 -> cfblk60/1
  cyemi_1385/1 -> cfblk61/1
  cyemi_1386/1 -> cfblk61/2
  cfblk140/1 -> cyemi_1386/1
  cyemi_1387/1 -> cfblk62/1
  cfblk217/1(cfblk2) -> cyemi_1387/1
  cyemi_1388/1 -> cfblk62/2
  cfblk201/2(cfblk12) -> cyemi_1388/1
  cyemi_1389/1 -> cfblk63/1
  cfblk2/1 -> cyemi_1389/1
  cyemi_1390/1 -> cfblk64/1
  cfblk141/1(Signal 1) -> cyemi_1390/1
  cyemi_1391/1 -> cfblk65/1
  cfblk142/1 -> cyemi_1391/1
  cyemi_1392/1 -> cfblk65/2
  cfblk227/2(cfblk12) -> cyemi_1392/1
  cyemi_1393/1 -> cfblk66/1
  cfblk72/1 -> cyemi_1393/1
  cyemi_1394/1 -> cfblk67/1
  cyemi_1395/1 -> cfblk68/1
  cfblk203/2(cfblk15) -> cyemi_1395/1
  cyemi_1396/1 -> cfblk69/1
  cyemi_1397/1 -> cfblk7/1
  cyemi_1398/1 -> cfblk70/1
  cfblk228/1(cfblk2) -> cyemi_1398/1
  cyemi_1399/1 -> cfblk71/1
  cfblk1/1 -> cyemi_1399/1
  cyemi_1400/1 -> cfblk72/1
  cfblk79/1 -> cyemi_1400/1
  cyemi_1401/1 -> cfblk73/1
  cfblk32/1 -> cyemi_1401/1
  cyemi_1402/1 -> cfblk74/1
  cfblk80/1 -> cyemi_1402/1
  cyemi_1403/1 -> cfblk75/1
  cfblk131/1 -> cyemi_1403/1
  cyemi_1404/1 -> cfblk75/2
  cyemi_1405/1 -> cfblk76/1
  cfblk21/1 -> cyemi_1405/1
  cyemi_1406/1 -> cfblk77/1
  cfblk59/1 -> cyemi_1406/1
  cyemi_1407/1 -> cfblk77/2
  cfblk208/2(cfblk7) -> cyemi_1407/1
  cyemi_1408/1 -> cfblk78/1
  cfblk13/1 -> cyemi_1408/1
  cyemi_1409/1 -> cfblk79/1
  cfblk83/1 -> cyemi_1409/1
  cyemi_1410/1 -> cfblk8/1
  cfblk23/1 -> cyemi_1410/1
  cyemi_1411/1 -> cfblk80/1
  cfblk242/3(cfblk15) -> cyemi_1411/1
  cyemi_1412/1 -> cfblk81/1
  cfblk218/3(cfblk17) -> cyemi_1412/1
  cyemi_1413/1 -> cfblk82/1
  cfblk156/1(Signal 1) -> cyemi_1413/1
  cyemi_1414/1 -> cfblk83/1
  cfblk19/1 -> cyemi_1414/1
  cyemi_1415/1 -> cfblk83/2
  cyemi_1416/1 -> cfblk88/1
  cfblk201/3(cfblk13) -> cyemi_1416/1
  cyemi_1417/1 -> cfblk9/1
  cfblk12/1 -> cyemi_1417/1
  cyemi_1418/1 -> cfblk94/1
  cfblk135/1 -> cyemi_1418/1
  cyemi_1419/1 -> cfblk96/1
  cfblk220/1(cfblk2) -> cyemi_1419/1
  cyemi_949/1 -> cyemi_1404/1, cyemi_1375/1
  cyemi_950/1 -> cyemi_1334/1
  cyemi_695/1 -> cyemi_1085/1
  cyemi_588/1 -> cyemi_634/1
  cyemi_393/1 -> cyemi_1296/1, cyemi_1369/1, cyemi_1323/1, cyemi_1353/1, cyemi_899/1
  cyemi_432/1 -> cyemi_37/1
  cyemi_658/1 -> cyemi_1394/1

== system sampleModel2432_pp_1_1/cfblk141 ==
  Demux : Demux  Tag=STV Demux  Outputs=1
  FromWs : FromWorkspace  Tag=STV FromWs  VariableName=tuvar  SampleTime=0
      SigBuilderData=|
      | common.afterFinalStr = 'Extrapolate'
      | common.sampleTime = 0
      | dataSet.timeRange = [0 10]
      | dataSet.name = 'Group 1'
      | sbobj.Groups.Name = 'Group 1'
      | sbobj.Groups.Signals.Name = 'Signal 1'
      | sbobj.Groups.Signals.XData = [0 4 4 6 6 10]
      | sbobj.Groups.Signals.YData = [0 0 1 1 0 0]
  Signal 1 : Outport  Tag=STV Outport
  wires:
  Demux/1 -> Signal 1/1
  FromWs/1 -> Demux/1

== system sampleModel2432_pp_1_1/cfblk156 ==
  Demux : Demux  Tag=STV Demux  Outputs=1
  FromWs : FromWorkspace  Tag=STV FromWs  VariableName=tuvar  SampleTime=0
      SigBuilderData=|
      | common.afterFinalStr = 'Extrapolate'
      | common.sampleTime = 0
      | dataSet.timeRange = [0 10]
      | dataSet.name = 'Group 1'
      | sbobj.Groups.Name = 'Group 1'
      | sbobj.Groups.Signals.Name = 'Signal 1'
      | sbobj.Groups.Signals.XData = [0 4 4 6 6 10]
      | sbobj.Groups.Signals.YData = [0 0 1 1 0 0]
  Signal 1 : Outport  Tag=STV Outport
  wires:
  Demux/1 -> Signal 1/1
  FromWs/1 -> Demux/1

== system sampleModel2432_pp_1_1/cfblk195 ==
  cfblk1 : Inport
  Action Port : ActionPort  ActionType=then
  cfblk3 : Delay  DelayLengthSource=Input port
      settings: InputPortMap=u0,p1
  cfblk4 : DiscreteStateSpace  SampleTime=-1
  cfblk5 : DiscreteFilter
  cfblk6 : simulink/Continuous/PID Controller (2DOF)  Controller=PID  TimeDomain=Discrete-time  SampleTime=-1  IntegratorMethod=Forward Euler  FilterMethod=Forward Euler  Form=Parallel  UseFilter=on  ControllerParametersSource=internal  P=1  I=1  D=0  N=100  b=1  c=1  InitialConditionSource=internal  InitialConditionForIntegrator=0  InitialConditionForFilter=0  ExternalReset=none  LimitOutput=off  UpperSaturationLimit=inf  LowerSaturationLimit=-inf  LinearizeAsGain=off  AntiWindupMode=none  Kb=1  TrackingMode=off  Kt=1  PParamMin=[]  PParamMax=[]  IParamMin=[]  IParamMax=[]  DParamMin=[]  DParamMax=[]  NParamMin=[]  NParamMax=[]  bParamMin=[]  bParamMax=[]  cParamMin=[]  cParamMax=[]  KbParamMin=[]  KbParamMax=[]  KtParamMin=[]  KtParamMax=[]  POutMin=[]  POutMax=[]  IOutMin=[]  IOutMax=[]  DOutMin=[]  DOutMax=[]  NOutMin=[]  NOutMax=[]  bOutMin=[]  bOutMax=[]  cOutMin=[]  cOutMax=[]  KbOutMin=[]  KbOutMax=[]  KtOutMin=[]  KtOutMax=[]  IntegratorOutMin=[]  IntegratorOutMax=[]  FilterOutMin=[]  FilterOutMax=[]  SumOutMin=[]  SumOutMax=[]  Sum1OutMin=[]  Sum1OutMax=[]  Sum2OutMin=[]  Sum2OutMax=[]  Sum3OutMin=[]  Sum3OutMax=[]  SumI1OutMin=[]  SumI1OutMax=[]  SumI2OutMin=[]  SumI2OutMax=[]  SumI3OutMin=[]  SumI3OutMax=[]  SumDOutMin=[]  SumDOutMax=[]  SaturationOutMin=[]  SaturationOutMax=[]  IntegratorContinuousStateAttributes=''  IntegratorStateMustResolveToSignalObject=off  IntegratorRTWStateStorageClass=Auto  FilterContinuousStateAttributes=''  FilterStateMustResolveToSignalObject=off  FilterRTWStateStorageClass=Auto  DifferentiatorICPrevScaledInput=0  DifferentiatorOutMin=[]  DifferentiatorOutMax=[]  FilterDiffOutCoefMin=[]  FilterDiffOutCoefMax=[]  SumDenOutMin=[]  SumDenOutMax=[]  SumNumOutMin=[]  SumNumOutMax=[]  ReciprocalOutMin=[]  ReciprocalOutMax=[]  DivideOutMin=[]  DivideOutMax=[]  TunerSelectOption=Transfer Function Based (PID Tuner App)
  cfblk8 : Delay
  cyemi_{48..54} (7 alike) : DataTypeConversion  OutDataTypeStr=double
  cfblk2 : Outport
  cfblk7 : Outport  Port=2
  wires:
  cfblk3/1 -> cfblk2/1, cyemi_51/1
  cfblk6/1 -> cfblk7/1, cyemi_49/1
  cyemi_48/1 -> cfblk3/1
  cfblk8/1 -> cyemi_48/1
  cyemi_49/1 -> cfblk3/2
  cyemi_50/1 -> cfblk4/1
  cfblk5/1 -> cyemi_50/1
  cyemi_51/1 -> cfblk5/1
  cyemi_52/1 -> cfblk6/1
  cfblk1/1 -> cyemi_52/1, cyemi_53/1
  cyemi_53/1 -> cfblk6/2
  cyemi_54/1 -> cfblk8/1
  cfblk4/1 -> cyemi_54/1

== system sampleModel2432_pp_1_1/cfblk196 ==
  cfblk1 : Inport
  Action Port : ActionPort  ActionType=else
  cfblk{10,14..17} (5 alike) : Delay
  cfblk11 : If  SampleTime=1
  cfblk12 : Subsystem  TreatAsAtomicUnit=on
  cfblk13 : Subsystem  TreatAsAtomicUnit=on
  cfblk3 : DiscreteFir
  cfblk4 : DiscreteTransferFcn
  cfblk5 : simulink/Discrete/Tapped Delay  vinit=0.0  samptime=-1  NumDelays=1  DelayOrder=Oldest  includeCurrent=off
  cfblk6 : DiscreteFilter
  cfblk7 : DiscreteIntegrator  SampleTime=-1  ICPrevOutput=DiscIntNeverNeededParam  ICPrevScaledInput=DiscIntNeverNeededParam
  cfblk8 : simulink/Discrete/Transfer Fcn Real Zero  ZeroZ=0.75  ICPrevInput=0.0  DoSatur=off
      settings: SourceProductName=Simulink  SourceProductBaseCode=SL
  cfblk9 : Delay  DelayLengthSource=Input port
      settings: InputPortMap=u0,p1
  cyemi_{56..59,69..70,77..88} (18 alike) : DataTypeConversion  OutDataTypeStr=double
  cfblk2 : Outport
  wires:
  cfblk9/1 -> cfblk2/1
  cfblk12/3(cfblk12) -> cyemi_83/1, cyemi_84/1
  cfblk11/1 -> cfblk12/Action
  cfblk11/2 -> cfblk13/Action
  cyemi_56/1 -> cfblk10/1
  cfblk8/1 -> cyemi_56/1
  cyemi_57/1 -> cfblk11/1
  cfblk14/1 -> cyemi_57/1
  cyemi_58/1 -> cfblk12/1(cfblk1)
  cfblk1/1 -> cyemi_58/1
  cyemi_59/1 -> cfblk12/2(cfblk10)
  cfblk17/1 -> cyemi_59/1
  cyemi_69/1 -> cfblk13/1(cfblk1)
  cfblk16/1 -> cyemi_69/1
  cyemi_70/1 -> cfblk13/2(cfblk8)
  cfblk15/1 -> cyemi_70/1
  cyemi_77/1 -> cfblk14/1
  cfblk10/1 -> cyemi_77/1
  cyemi_78/1 -> cfblk15/1
  cfblk3/1 -> cyemi_78/1
  cyemi_79/1 -> cfblk16/1
  cfblk7/1 -> cyemi_79/1
  cyemi_80/1 -> cfblk17/1
  cfblk5/1 -> cyemi_80/1
  cyemi_81/1 -> cfblk3/1
  cfblk13/1(cfblk2) -> cyemi_81/1
  cyemi_82/1 -> cfblk4/1
  cfblk12/1(cfblk2) -> cyemi_82/1
  cyemi_83/1 -> cfblk5/1
  cyemi_84/1 -> cfblk6/1
  cyemi_85/1 -> cfblk7/1
  cfblk13/2(cfblk9) -> cyemi_85/1
  cyemi_86/1 -> cfblk8/1
  cfblk4/1 -> cyemi_86/1
  cyemi_87/1 -> cfblk9/1
  cfblk6/1 -> cyemi_87/1
  cyemi_88/1 -> cfblk9/2
  cfblk12/2(cfblk11) -> cyemi_88/1

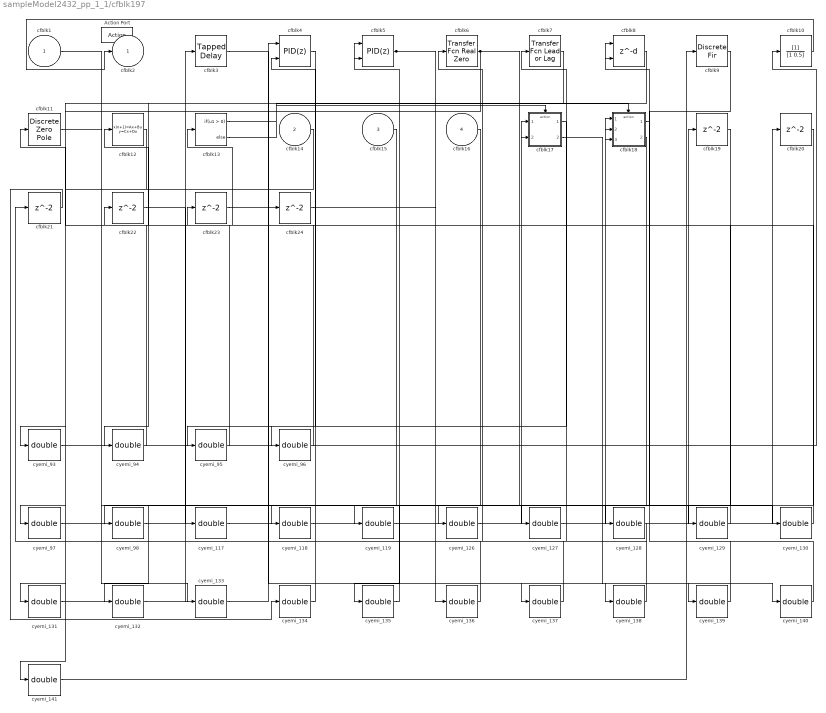
== system sampleModel2432_pp_1_1/cfblk197 ==
  cfblk1 : Inport
  cfblk14 : Inport  Port=2
  cfblk15 : Inport  Port=3
  cfblk16 : Inport  Port=4
  Action Port : ActionPort  ActionType=then
  cfblk10 : DiscreteFilter
  cfblk11 : DiscreteZeroPole  Poles=[0 0.5]  Gain=1  SampleTime=-1
  cfblk12 : DiscreteStateSpace  SampleTime=-1
  cfblk13 : If  SampleTime=1
  cfblk17 : Subsystem  TreatAsAtomicUnit=on
  cfblk18 : Subsystem  TreatAsAtomicUnit=on
  cfblk{19..24} (6 alike) : Delay
  cfblk3 : simulink/Discrete/Tapped Delay  vinit=0.0  samptime=-1  NumDelays=1  DelayOrder=Oldest  includeCurrent=off
  cfblk4 : simulink/Continuous/PID Controller (2DOF)  Controller=PID  TimeDomain=Discrete-time  SampleTime=-1  IntegratorMethod=Forward Euler  FilterMethod=Forward Euler  Form=Parallel  UseFilter=on  ControllerParametersSource=internal  P=1  I=1  D=0  N=100  b=1  c=1  InitialConditionSource=internal  InitialConditionForIntegrator=0  InitialConditionForFilter=0  ExternalReset=none  LimitOutput=off  UpperSaturationLimit=inf  LowerSaturationLimit=-inf  LinearizeAsGain=off  AntiWindupMode=none  Kb=1  TrackingMode=off  Kt=1  PParamMin=[]  PParamMax=[]  IParamMin=[]  IParamMax=[]  DParamMin=[]  DParamMax=[]  NParamMin=[]  NParamMax=[]  bParamMin=[]  bParamMax=[]  cParamMin=[]  cParamMax=[]  KbParamMin=[]  KbParamMax=[]  KtParamMin=[]  KtParamMax=[]  POutMin=[]  POutMax=[]  IOutMin=[]  IOutMax=[]  DOutMin=[]  DOutMax=[]  NOutMin=[]  NOutMax=[]  bOutMin=[]  bOutMax=[]  cOutMin=[]  cOutMax=[]  KbOutMin=[]  KbOutMax=[]  KtOutMin=[]  KtOutMax=[]  IntegratorOutMin=[]  IntegratorOutMax=[]  FilterOutMin=[]  FilterOutMax=[]  SumOutMin=[]  SumOutMax=[]  Sum1OutMin=[]  Sum1OutMax=[]  Sum2OutMin=[]  Sum2OutMax=[]  Sum3OutMin=[]  Sum3OutMax=[]  SumI1OutMin=[]  SumI1OutMax=[]  SumI2OutMin=[]  SumI2OutMax=[]  SumI3OutMin=[]  SumI3OutMax=[]  SumDOutMin=[]  SumDOutMax=[]  SaturationOutMin=[]  SaturationOutMax=[]  IntegratorContinuousStateAttributes=''  IntegratorStateMustResolveToSignalObject=off  IntegratorRTWStateStorageClass=Auto  FilterContinuousStateAttributes=''  FilterStateMustResolveToSignalObject=off  FilterRTWStateStorageClass=Auto  DifferentiatorICPrevScaledInput=0  DifferentiatorOutMin=[]  DifferentiatorOutMax=[]  FilterDiffOutCoefMin=[]  FilterDiffOutCoefMax=[]  SumDenOutMin=[]  SumDenOutMax=[]  SumNumOutMin=[]  SumNumOutMax=[]  ReciprocalOutMin=[]  ReciprocalOutMax=[]  DivideOutMin=[]  DivideOutMax=[]  TunerSelectOption=Transfer Function Based (PID Tuner App)
  cfblk5 : simulink/Continuous/PID Controller (2DOF)  Controller=PID  TimeDomain=Discrete-time  SampleTime=-1  IntegratorMethod=Forward Euler  FilterMethod=Forward Euler  Form=Parallel  UseFilter=on  ControllerParametersSource=internal  P=1  I=1  D=0  N=100  b=1  c=1  InitialConditionSource=internal  InitialConditionForIntegrator=0  InitialConditionForFilter=0  ExternalReset=none  LimitOutput=off  UpperSaturationLimit=inf  LowerSaturationLimit=-inf  LinearizeAsGain=off  AntiWindupMode=none  Kb=1  TrackingMode=off  Kt=1  PParamMin=[]  PParamMax=[]  IParamMin=[]  IParamMax=[]  DParamMin=[]  DParamMax=[]  NParamMin=[]  NParamMax=[]  bParamMin=[]  bParamMax=[]  cParamMin=[]  cParamMax=[]  KbParamMin=[]  KbParamMax=[]  KtParamMin=[]  KtParamMax=[]  POutMin=[]  POutMax=[]  IOutMin=[]  IOutMax=[]  DOutMin=[]  DOutMax=[]  NOutMin=[]  NOutMax=[]  bOutMin=[]  bOutMax=[]  cOutMin=[]  cOutMax=[]  KbOutMin=[]  KbOutMax=[]  KtOutMin=[]  KtOutMax=[]  IntegratorOutMin=[]  IntegratorOutMax=[]  FilterOutMin=[]  FilterOutMax=[]  SumOutMin=[]  SumOutMax=[]  Sum1OutMin=[]  Sum1OutMax=[]  Sum2OutMin=[]  Sum2OutMax=[]  Sum3OutMin=[]  Sum3OutMax=[]  SumI1OutMin=[]  SumI1OutMax=[]  SumI2OutMin=[]  SumI2OutMax=[]  SumI3OutMin=[]  SumI3OutMax=[]  SumDOutMin=[]  SumDOutMax=[]  SaturationOutMin=[]  SaturationOutMax=[]  IntegratorContinuousStateAttributes=''  IntegratorStateMustResolveToSignalObject=off  IntegratorRTWStateStorageClass=Auto  FilterContinuousStateAttributes=''  FilterStateMustResolveToSignalObject=off  FilterRTWStateStorageClass=Auto  DifferentiatorICPrevScaledInput=0  DifferentiatorOutMin=[]  DifferentiatorOutMax=[]  FilterDiffOutCoefMin=[]  FilterDiffOutCoefMax=[]  SumDenOutMin=[]  SumDenOutMax=[]  SumNumOutMin=[]  SumNumOutMax=[]  ReciprocalOutMin=[]  ReciprocalOutMax=[]  DivideOutMin=[]  DivideOutMax=[]  TunerSelectOption=Transfer Function Based (PID Tuner App)
  cfblk6 : simulink/Discrete/Transfer Fcn Real Zero  ZeroZ=0.75  ICPrevInput=0.0  DoSatur=off
      settings: SourceProductName=Simulink  SourceProductBaseCode=SL
  cfblk7 : simulink/Discrete/Transfer Fcn Lead or Lag  PoleZ=0.95  ZeroZ=0.75  ICPrevOutput=0.0  ICPrevInput=0.0  DoSatur=off
      settings: SourceProductName=Simulink  SourceProductBaseCode=SL
  cfblk8 : Delay  DelayLengthSource=Input port
      settings: InputPortMap=u0,p1
  cfblk9 : DiscreteFir
  cyemi_{93..98,117..119,126..141} (25 alike) : DataTypeConversion  OutDataTypeStr=double
  cfblk2 : Outport
  wires:
  cfblk5/1 -> cyemi_129/1, cyemi_137/1
  cfblk6/1 -> cyemi_130/1, cyemi_131/1
  cfblk10/1 -> cfblk2/1
  cfblk13/1 -> cfblk17/Action
  cfblk13/2 -> cfblk18/Action
  cyemi_93/1 -> cfblk10/1
  cfblk14/1 -> cyemi_93/1
  cyemi_94/1 -> cfblk11/1
  cfblk8/1 -> cyemi_94/1
  cyemi_95/1 -> cfblk12/1
  cfblk17/1(cfblk2) -> cyemi_95/1
  cyemi_96/1 -> cfblk13/1
  cfblk4/1 -> cyemi_96/1
  cyemi_97/1 -> cfblk17/1(cfblk1)
  cfblk7/1 -> cyemi_97/1
  cyemi_98/1 -> cfblk17/2(cfblk16)
  cfblk19/1 -> cyemi_98/1
  cyemi_117/1 -> cfblk18/1(cfblk1)
  cfblk22/1 -> cyemi_117/1
  cyemi_118/1 -> cfblk18/2(cfblk9)
  cfblk20/1 -> cyemi_118/1
  cyemi_119/1 -> cfblk18/3(cfblk10)
  cfblk15/1 -> cyemi_119/1
  cyemi_126/1 -> cfblk19/1
  cfblk9/1 -> cyemi_126/1
  cyemi_127/1 -> cfblk20/1
  cfblk11/1 -> cyemi_127/1
  cyemi_128/1 -> cfblk21/1
  cfblk18/1(cfblk2) -> cyemi_128/1
  cyemi_129/1 -> cfblk22/1
  cyemi_130/1 -> cfblk23/1
  cyemi_131/1 -> cfblk24/1
  cyemi_132/1 -> cfblk3/1
  cfblk16/1 -> cyemi_132/1
  cyemi_133/1 -> cfblk4/1
  cfblk1/1 -> cyemi_133/1
  cyemi_134/1 -> cfblk4/2
  cfblk21/1 -> cyemi_134/1
  cyemi_135/1 -> cfblk5/1
  cfblk18/2(cfblk11) -> cyemi_135/1
  cyemi_136/1 -> cfblk5/2
  cfblk24/1 -> cyemi_136/1
  cyemi_137/1 -> cfblk6/1
  cyemi_138/1 -> cfblk7/1
  cfblk3/1 -> cyemi_138/1
  cyemi_139/1 -> cfblk8/1
  cfblk23/1 -> cyemi_139/1
  cyemi_140/1 -> cfblk8/2
  cfblk17/2(cfblk17) -> cyemi_140/1
  cyemi_141/1 -> cfblk9/1
  cfblk12/1 -> cyemi_141/1

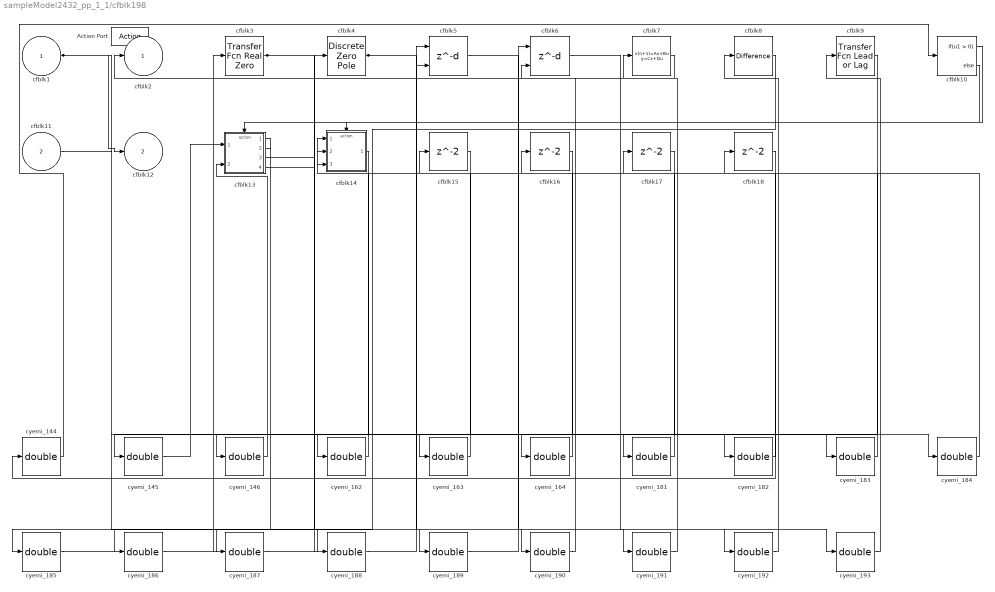
== system sampleModel2432_pp_1_1/cfblk198 ==
  cfblk1 : Inport
  cfblk11 : Inport  Port=2
  Action Port : ActionPort  ActionType=else
  cfblk10 : If  SampleTime=1
  cfblk13 : Subsystem  TreatAsAtomicUnit=on
  cfblk14 : Subsystem  TreatAsAtomicUnit=on
  cfblk{15..18} (4 alike) : Delay
  cfblk3 : simulink/Discrete/Transfer Fcn Real Zero  ZeroZ=0.75  ICPrevInput=0.0  DoSatur=off
      settings: SourceProductName=Simulink  SourceProductBaseCode=SL
  cfblk4 : DiscreteZeroPole  Poles=[0 0.5]  Gain=1  SampleTime=-1
  cfblk5 : Delay  DelayLengthSource=Input port
      settings: InputPortMap=u0,p1
  cfblk6 : Delay  DelayLengthSource=Input port
      settings: InputPortMap=u0,p1
  cfblk7 : DiscreteStateSpace  SampleTime=-1
  cfblk8 : simulink/Discrete/Difference  ICPrevInput=0.0  OutMin=[]  OutMax=[]  OutDataTypeStr=Inherit: Inherit via back propagation  OutDataType=fixdt(1, 16)  OutScaling=2^-10  DoSatur=off
  cfblk9 : simulink/Discrete/Transfer Fcn Lead or Lag  PoleZ=0.95  ZeroZ=0.75  ICPrevOutput=0.0  ICPrevInput=0.0  DoSatur=off
      settings: SourceProductName=Simulink  SourceProductBaseCode=SL
  cyemi_{144..146,162..164,181..193} (19 alike) : DataTypeConversion  OutDataTypeStr=double
  cfblk2 : Outport
  cfblk12 : Outport  Port=2
  wires:
  cfblk3/1 -> cyemi_182/1, cyemi_189/1
  cfblk7/1 -> cfblk2/1
  cfblk1/1 -> cfblk12/1, cyemi_162/1
  cfblk4/1 -> cyemi_183/1, cyemi_191/1
  cfblk10/1 -> cfblk13/Action
  cfblk10/2 -> cfblk14/Action
  cyemi_144/1 -> cfblk10/1
  cfblk18/1 -> cyemi_144/1
  cyemi_145/1 -> cfblk13/1(cfblk1)
  cfblk14/1(cfblk2) -> cyemi_145/1
  cyemi_146/1 -> cfblk13/2(cfblk13)
  cfblk15/1 -> cyemi_146/1
  cyemi_162/1 -> cfblk14/1(cfblk1)
  cyemi_163/1 -> cfblk14/2(cfblk11)
  cfblk17/1 -> cyemi_163/1
  cyemi_164/1 -> cfblk14/3(cfblk12)
  cfblk16/1 -> cyemi_164/1
  cyemi_181/1 -> cfblk15/1
  cfblk9/1 -> cyemi_181/1
  cyemi_182/1 -> cfblk16/1
  cyemi_183/1 -> cfblk17/1
  cyemi_184/1 -> cfblk18/1
  cfblk13/3(cfblk15) -> cyemi_184/1
  cyemi_185/1 -> cfblk3/1
  cfblk13/1(cfblk2) -> cyemi_185/1
  cyemi_186/1 -> cfblk4/1
  cfblk13/2(cfblk14) -> cyemi_186/1
  cyemi_187/1 -> cfblk5/1
  cfblk8/1 -> cyemi_187/1
  cyemi_188/1 -> cfblk5/2
  cfblk11/1 -> cyemi_188/1
  cyemi_189/1 -> cfblk6/1
  cyemi_190/1 -> cfblk6/2
  cfblk13/4(cfblk16) -> cyemi_190/1
  cyemi_191/1 -> cfblk7/1
  cyemi_192/1 -> cfblk8/1
  cfblk6/1 -> cyemi_192/1
  cyemi_193/1 -> cfblk9/1
  cfblk5/1 -> cyemi_193/1

== system sampleModel2432_pp_1_1/cfblk199 ==
  cfblk1 : Inport
  Action Port : ActionPort  ActionType=then
  cfblk10 : Delay  DelayLengthSource=Input port
      settings: InputPortMap=u0,p1
  cfblk3 : DiscreteFilter
  cfblk4 : DiscreteIntegrator  SampleTime=-1  ICPrevOutput=DiscIntNeverNeededParam  ICPrevScaledInput=DiscIntNeverNeededParam
  cfblk5 : Delay  ShowEnablePort=on
      settings: InputPortMap=u0,e6
  cfblk6 : simulink/Discrete/Transfer Fcn First Order  PoleZ=0.95  ICPrevOutput=0.0  DoSatur=off
      settings: SourceProductName=Simulink
  cfblk7 : simulink/Discrete/Tapped Delay  vinit=0.0  samptime=-1  NumDelays=1  DelayOrder=Oldest  includeCurrent=off
  cfblk8 : UnitDelay  SampleTime=-1
  cfblk9 : DiscreteZeroPole  Poles=[0 0.5]  Gain=1  SampleTime=-1
  cyemi_{195..204} (10 alike) : DataTypeConversion  OutDataTypeStr=double
  cfblk2 : Outport
  cfblk11 : Outport  Port=2
  wires:
  cfblk6/1 -> cyemi_198/1, cyemi_202/1
  cfblk4/1 -> cfblk11/1, cyemi_196/1, cyemi_200/1
  cfblk3/1 -> cfblk2/1
  cyemi_195/1 -> cfblk10/1
  cfblk8/1 -> cyemi_195/1
  cyemi_196/1 -> cfblk10/2
  cyemi_197/1 -> cfblk3/1
  cfblk5/1 -> cyemi_197/1
  cyemi_198/1 -> cfblk4/1
  cyemi_199/1 -> cfblk5/1
  cfblk9/1 -> cyemi_199/1
  cyemi_200/1 -> cfblk5/2
  cyemi_201/1 -> cfblk6/1
  cfblk1/1 -> cyemi_201/1
  cyemi_202/1 -> cfblk7/1
  cyemi_203/1 -> cfblk8/1
  cfblk7/1 -> cyemi_203/1
  cyemi_204/1 -> cfblk9/1
  cfblk10/1 -> cyemi_204/1

== system sampleModel2432_pp_1_1/cfblk200 ==
  cfblk1 : Inport
  cfblk8 : Inport  Port=2
  cfblk9 : Inport  Port=3
  Action Port : ActionPort  ActionType=else
  cfblk11 : Delay
  cfblk3 : UnitDelay  SampleTime=-1
  cfblk4 : DiscreteTransferFcn
  cfblk5 : DiscreteFilter
  cfblk6 : DiscreteFir
  cfblk7 : simulink/Discrete/Tapped Delay  vinit=0.0  samptime=-1  NumDelays=1  DelayOrder=Oldest  includeCurrent=off
  cyemi_{210..215} (6 alike) : DataTypeConversion  OutDataTypeStr=double
  cfblk2 : Outport
  cfblk10 : Outport  Port=2
  wires:
  cfblk8/1 -> cfblk2/1
  cfblk5/1 -> cfblk10/1
  cyemi_210/1 -> cfblk11/1
  cfblk7/1 -> cyemi_210/1
  cyemi_211/1 -> cfblk3/1
  cfblk11/1 -> cyemi_211/1
  cyemi_212/1 -> cfblk4/1
  cfblk6/1 -> cyemi_212/1
  cyemi_213/1 -> cfblk5/1
  cfblk4/1 -> cyemi_213/1
  cyemi_214/1 -> cfblk6/1
  cfblk9/1 -> cyemi_214/1
  cyemi_215/1 -> cfblk7/1
  cfblk3/1 -> cyemi_215/1
